simulink model "ThomasJana_WorkingCode (fix branch)"  (R2023a)
settings: Solver=FixedStepDiscrete  StartTime=0.0  StopTime=inf  FixedStep=0.0001  RelTol=1e-3
undefined symbols (not defined in the file): DiscIntNeverNeededParam
libraries: arduinolib x13, simulink x3, hdlsllib x2, slpidlib x1, mobileRoboticsTrainingLib x1, arduinosensorlib x1
(part 2 of 2)

== stateflow chart ThomasJana_WorkingCode (fix branch)/Motion Control1/Intersection Navigation V2 ==
  note: Basic Description
      | Default: Curve Navigation controls the velocity and angular velocity
      |
      | When infrared sensor 1 or 4 (IR1 and IR4) detect a black line, this Intersection Navigation subsystem takes control and calls the leftTurn or rightTurn procedure respectively.
      | Intersection procedure (same for both leftTurn or rightTurn):
      | 	Increment branchCounter to keep track of the number of branches.
      | 	Move forward a small distance to align with the turn.
      | 	Rotate in the correct direction until the middle two sensors detect a line again.
      | 	Pass control to Curve Navigation to navigate the offshoot.
      | 	If the offshoot comes to an end (all sensors detect white), rotate 180 degrees and navigate back to the main path.
      | 	If the offshoot ends in a detect line (all sensors detect black), stop, send a signal to the Object Detection subsystem to measure for an object, rotate 180 degrees and navigate back to the main path.
      | 		Add branch number from branchCounter to objectMap to indicate this branch has an object.
      | 	Pass control to Curve Navigation to navigate the offshoot returning to the main path.
      | 	When the peripheral sensors detect a black line again (meaning the robot has returned to the intersection with the main branch), control is passed to Intersection Navigation.
      | 	Move forward a small distance to align with the turn.
      | 	Rotate in the correct direction until the middle two sensors detect a line again.
      | 	Pass control back to Curve Navigation to continue traversing the main path.
      |
      | If all sensors detect black whilst the robot is on the main path, the endOfMaze procedure is called.
      | endOfMaze procedure:
      | 	Stop
      | 	Use objectMap to determine how many objects were discovered.
      | 	Find the branch number of the object with the smallest distance, saved to branchWithObject.
      | 		objectCounter provides number of object with smallest distance measured.
      | 		Obtain the n'th number in objectMap to determine the branch number containing said object (where n = objectCounter)
      | 	Invert branchWithObject such that it provides the number of the branch starting from the end of the maze.
      | 	Set renavigating to HIGH.
      |
      | Renavigating Procedure:
      | 	Rotate 180 degrees to re-traverse the maze.
      | 	set branchCounter to 0.
      | 	Pass control to Curve Navigation to renavigate maze.
      | 	If intersection is detected, increment branchCounter.
      | 	If branchCounter is equal to branchWithObject at an intersection, turn into that offshoot.
      | 	Pass control to Curve Navigation to navigate offshoot.
      | 	If all sensors detect black at the "detect object line", come to a stop.
  note: Note to self:
      | Make sure all blocks with forward velocity use curve-following algorithm (never move forward blindly)
      |
      | Neaten up blocks
      |
      | Add 4way navigation
      |
      | Make back and forth smaller (will need to be adjusted for real life speed)
  state analyseIntersection
    state returnToIntersection
      entry: distance0 = distance;
      state FollowTrack
        %middle two sense black
        velocity = -0.5;
        angular_velocity = 0;
      state TurnLeft
        entry:
        velocity = 0;
        angular_velocity = 2;
      state TurnRight
        entry:
        velocity = 0;
        angular_velocity = -2;
      (default) -> analyseIntersection.returnToIntersection.FollowTrack
      analyseIntersection.returnToIntersection.TurnRight -> analyseIntersection.returnToIntersection.FollowTrack : [IR3 == 0 && IR2 == 0]
      analyseIntersection.returnToIntersection.TurnLeft -> analyseIntersection.returnToIntersection.FollowTrack : [IR3 == 0 && IR2 == 0]
      analyseIntersection.returnToIntersection.FollowTrack -> analyseIntersection.returnToIntersection.TurnRight [order 2] : [IR2 == 1]
      analyseIntersection.returnToIntersection.FollowTrack -> analyseIntersection.returnToIntersection.TurnLeft [order 1] : [IR3 == 1]
    state moveForward
      entry: distance0 = distance;
      state FollowTrack
        %middle two sense black
        velocity = 1;
        angular_velocity = 0;
      state TurnLeft
        entry:
        velocity = 0;
        angular_velocity = -2;
      state TurnRight
        entry:
        velocity = 0;
        angular_velocity = 2;
      analyseIntersection.moveForward.FollowTrack -> analyseIntersection.moveForward.TurnLeft [order 1] : [IR3 == 1]
      analyseIntersection.moveForward.TurnRight -> analyseIntersection.moveForward.FollowTrack : [IR3 == 0 && IR2 == 0]
      analyseIntersection.moveForward.FollowTrack -> analyseIntersection.moveForward.TurnRight [order 2] : [IR2 == 1]
      analyseIntersection.moveForward.TurnLeft -> analyseIntersection.moveForward.FollowTrack : [IR3 == 0 && IR2 == 0]
      (default) -> analyseIntersection.moveForward.FollowTrack
    state chooseIntersectionType
      %left turn
      %extreme left turn
      %right turn
      %extreme right turn
      %end of maze
      %4-way junction
      entry: velocity = 0;
      angular_velocity = 0;
    state commenceIntersectionControl
      entry: velocity = 0;
    (default) -> analyseIntersection.moveForward
    chooseIntersectionType -> returnToIntersection [order 1] : [(IR2 == 0 || IR3 == 0)]
    returnToIntersection -> commenceIntersectionControl : [IR1 == 0 || IR4 == 0]
    (junction 486) -> returnToIntersection : {finishMaze = 1;}
    analyseIntersection.moveForward -> chooseIntersectionType : [IR1 == 1 && IR4 == 1]
    chooseIntersectionType -> (junction 486) [order 3] : [IR1 + IR2 + IR3 + IR4 == 4]{fourWay = 0;}
    chooseIntersectionType -> (junction 486) [order 2] : [IR1 + IR2 + IR3 + IR4 == 0]{fourWay = 0;}
  note: if fourway doesn't work now:
      | have it pick up if another intersection is ever picked up in the slight move forward, and then limit forward movement massivly.
      | If another interesction in opposite direction was ever picked up - four way
  state endOfMaze
    %procedure to locate position of closest object once maze is completed
    entry: velocity = 0;
    angular_velocity = 0;
    num = objectMap;
    while num > 0
    len = len + 1;
    num = fix(num/10);
    end
    branchWithObject = mod(fix(objectMap/10^(len - objectCounter)), 10);
    branchWithObject = branchCounter - branchWithObject + 1
    exit:
    renavigating = 1;
  state fullRotation
    %rotate 180 degrees to renavigate maze
    entry: phi0 = phi;
    during:
    velocity = 0;
    angular_velocity = -1;
  note: if fullInter == 1:
      | if all black:
  state followMain
    state TurnRight
      entry:
      velocity = 0;
      angular_velocity = 2;
    state FollowTrack
      %middle two sense black
      velocity = 1;
      angular_velocity = 0;
    state TurnLeft
      entry:
      velocity = 0;
      angular_velocity = -2;
    (default) -> followMain.FollowTrack
    followMain.FollowTrack -> followMain.TurnLeft [order 2] : [IR3 == 1]
    followMain.TurnRight -> followMain.FollowTrack : [IR3 == 0 && IR2 == 0]
    followMain.TurnLeft -> followMain.FollowTrack : [IR3 == 0 && IR2 == 0]
    followMain.FollowTrack -> followMain.TurnRight [order 4] : [IR2 == 1]
    (junction 442) -> followMain.FollowTrack
    (junction 440) -> followMain.FollowTrack
  state Wait
  state leftTurn
    %procedure for navigating an offshoot to the right of the main path
    state Rotate
      entry:  branchCounter = branchCounter +1
      state moveForward
        entry: velocity = 1;
      state rotateOffPath
        entry:
        velocity = 0;
        angular_velocity = -1;
      state rotateOntoPath
      (default) -> leftTurn.Rotate.moveForward
      leftTurn.Rotate.moveForward -> leftTurn.Rotate.rotateOffPath : [IR1 == 1]
      leftTurn.Rotate.rotateOffPath -> (junction 365) : [IR2 == 1 && IR3 == 1]
      (junction 365) -> leftTurn.Rotate.rotateOntoPath
    state returnToMain
      state FollowTrack
        %middle two sense black
        velocity = 1;
        angular_velocity = 0;
      state TurnRight
        entry:
        velocity = 0;
        angular_velocity = 2;
      state TurnLeft1
        entry:
        velocity = 0;
        angular_velocity = -2;
      (default) -> leftTurn.returnToMain.FollowTrack
      (junction 469) -> leftTurn.returnToMain.FollowTrack
      (junction 472) -> leftTurn.returnToMain.FollowTrack
      TurnLeft1 -> (junction 469) : [IR3 == 0 && IR2 == 0]
      leftTurn.returnToMain.TurnRight -> (junction 472) : [IR3 == 0 && IR2 == 0]
      leftTurn.returnToMain.FollowTrack -> (junction 471) [order 2] : [IR2 == 1]
      leftTurn.returnToMain.FollowTrack -> (junction 470) [order 1] : [IR3 == 1]
      (junction 471) -> leftTurn.returnToMain.TurnRight
      (junction 470) -> TurnLeft1
    state leftToMain
      state moveForward
        entry: velocity = 1;
      state rotateOntoPath
      state rotateOffPath
        entry:
        velocity = 0;
        angular_velocity = 1;
      (default) -> leftTurn.leftToMain.moveForward
      leftTurn.leftToMain.moveForward -> leftTurn.leftToMain.rotateOffPath : [IR1 == 1]
      (junction 393) -> leftTurn.leftToMain.rotateOntoPath
      leftTurn.leftToMain.rotateOffPath -> (junction 393) : [IR2 == 1 && IR3 == 1]
    state navigateOffshoot
      state FollowTrack
        %middle two sense black
        velocity = 1;
        angular_velocity = 0;
      state TurnLeft
        entry:
        velocity = 0;
        angular_velocity = -2;
      state TurnRight
        entry:
        velocity = 0;
        angular_velocity = 2;
      (default) -> leftTurn.navigateOffshoot.FollowTrack
      leftTurn.navigateOffshoot.FollowTrack -> (junction 460) [order 2] : [IR2 == 1]
      (junction 460) -> leftTurn.navigateOffshoot.TurnRight
      leftTurn.navigateOffshoot.FollowTrack -> (junction 463) [order 1] : [IR3 == 1]
      (junction 463) -> leftTurn.navigateOffshoot.TurnLeft
      (junction 461) -> leftTurn.navigateOffshoot.FollowTrack : [IR3 == 0 && IR2 == 0]
      (junction 462) -> leftTurn.navigateOffshoot.FollowTrack
      leftTurn.navigateOffshoot.TurnRight -> (junction 461)
      leftTurn.navigateOffshoot.TurnLeft -> (junction 462) : [IR3 == 0 && IR2 == 0]
    state fullRotation
      %rotate 180 degrees
      entry: phi0 = phi;
      during:
      velocity = 0;
      angular_velocity = -4;
    state stopAndMeasure
      entry:
      velocity = 0;
      angular_velocity = 0;
      collectMeasurement = 1;
      exit:
      collectMeasurement = 0;
    state finalStop
      velocity = 0;
      angular_velocity = 0;
    (default) -> leftTurn.Rotate
    leftTurn.Rotate.rotateOntoPath -> leftTurn.navigateOffshoot : [IR2 == 0]
    leftTurn.returnToMain -> leftToMain : [IR1 == 0]
    leftTurn.fullRotation -> leftTurn.returnToMain : [abs(phi - phi0) > 2.793 && abs(phi - phi0) < 3.491 && IR2 == 0 && IR3 == 0]
    leftTurn.navigateOffshoot -> (junction 263) [order 2]
    (junction 263) -> (junction 264) : [IR1 + IR2 + IR3 + IR4 == 0 && renavigating == 1]
    leftTurn.navigateOffshoot -> (junction 216) [order 1] : [IR1 == 1 && IR2 == 1 && IR3 == 1 && IR4 == 1]
    (junction 216) -> leftTurn.fullRotation
    leftTurn.navigateOffshoot -> leftTurn.stopAndMeasure [order 3] : [IR1 == 0 && IR2 == 0 && IR3 == 0 && IR4 ==0]{objectMap = objectMap*10 + branchCounter;} %detect or stop line
    leftTurn.stopAndMeasure -> leftTurn.fullRotation : after(1, sec) [measurementComplete == 1]
    (junction 264) -> leftTurn.finalStop
  state rightTurn
    %procedure for navigating an offshoot to the right of the main path
    state returnToMain
      state FollowTrack
        %middle two sense black
        velocity = 1;
        angular_velocity = 0;
      state TurnLeft
        entry:
        velocity = 0;
        angular_velocity = -2;
      state TurnRight
        entry:
        velocity = 0;
        angular_velocity = 2;
      (default) -> rightTurn.returnToMain.FollowTrack
      rightTurn.returnToMain.FollowTrack -> rightTurn.returnToMain.TurnRight [order 2] : [IR2 == 1]
      rightTurn.returnToMain.TurnRight -> rightTurn.returnToMain.FollowTrack : [IR3 == 0 && IR2 == 0]
      rightTurn.returnToMain.FollowTrack -> rightTurn.returnToMain.TurnLeft [order 1] : [IR3 == 1]
      rightTurn.returnToMain.TurnLeft -> rightTurn.returnToMain.FollowTrack : [IR3 == 0 && IR2 == 0]
    state Rotate
      entry:  branchCounter = branchCounter +1
      state moveForward
        entry: velocity = 1;
      state rotateOffPath
        entry:
        velocity = 0;
        angular_velocity = 1;
      state rotateOntoPath
      (default) -> rightTurn.Rotate.moveForward
      rightTurn.Rotate.moveForward -> rightTurn.Rotate.rotateOffPath : [IR4 == 1]
      rightTurn.Rotate.rotateOffPath -> (junction 311) : [IR2 == 1 && IR3 == 1]
      (junction 311) -> rightTurn.Rotate.rotateOntoPath
    state rightToMain
      %turn right back onto the main path
      state moveForward
        entry: velocity = 1;
      state rotateOffPath
        entry:
        velocity = 0;
        angular_velocity = 1;
      state rotateOntoPath
      (default) -> rightTurn.rightToMain.moveForward
      rightTurn.rightToMain.moveForward -> rightTurn.rightToMain.rotateOffPath : [IR4 == 1]
      rightTurn.rightToMain.rotateOffPath -> (junction 357) : [IR2 == 1 && IR3 == 1]
      (junction 357) -> rightTurn.rightToMain.rotateOntoPath
    state navigateOffshoot
      state FollowTrack
        %middle two sense black
        velocity = 1;
        angular_velocity = 0;
      state TurnLeft
        entry:
        velocity = 0;
        angular_velocity = -2;
      state TurnRight1
        entry:
        velocity = 0;
        angular_velocity = 2;
      rightTurn.navigateOffshoot.FollowTrack -> (junction 448) [order 2] : [IR2 == 1]
      rightTurn.navigateOffshoot.FollowTrack -> (junction 454) [order 1] : [IR3 == 1]
      (junction 448) -> TurnRight1
      (junction 454) -> rightTurn.navigateOffshoot.TurnLeft
      (junction 450) -> rightTurn.navigateOffshoot.FollowTrack
      (default) -> rightTurn.navigateOffshoot.FollowTrack
      (junction 452) -> rightTurn.navigateOffshoot.FollowTrack
      TurnRight1 -> (junction 450) : [IR3 == 0 && IR2 == 0]
      rightTurn.navigateOffshoot.TurnLeft -> (junction 452) : [IR3 == 0 && IR2 == 0]
    state stopAndMeasure
      entry:
      velocity = 0;
      angular_velocity = 0;
      collectMeasurement = 1;
      exit:
      collectMeasurement = 0;
    state fullRotation
      %rotate 180 degrees
      entry: phi0 = phi;
      during:
      velocity = 0;
      angular_velocity = -4;
    state finalStop
      velocity = 0;
      angular_velocity = 0;
    (default) -> rightTurn.Rotate
    rightTurn.returnToMain -> rightToMain : [IR4 == 0]
    rightTurn.fullRotation -> rightTurn.returnToMain : [abs(phi - phi0) > 2.793 && abs(phi - phi0) < 3.491 && IR2 == 0 && IR3 == 0]
    rightTurn.Rotate.rotateOntoPath -> rightTurn.navigateOffshoot : [IR3 == 0]
    rightTurn.navigateOffshoot -> (junction 254) [order 1]
    (junction 254) -> (junction 256) : [IR1 + IR2 + IR3 + IR4 == 0 && renavigating == 1]
    rightTurn.navigateOffshoot -> (junction 194) [order 3] : [IR1 == 1 && IR2 == 1 && IR3 == 1 && IR4 == 1]
    (junction 194) -> rightTurn.fullRotation
    rightTurn.navigateOffshoot -> rightTurn.stopAndMeasure [order 2] : [IR1 == 0 && IR2 == 0 && IR3 == 0 && IR4 ==0]{objectMap = objectMap*10 + branchCounter;} %detect or stop line
    rightTurn.stopAndMeasure -> rightTurn.fullRotation : after(1, sec) [measurementComplete == 1]
    (junction 256) -> rightTurn.finalStop
  state renavigatingCounter
    entry:
    branchCounter = branchCounter + 1;
  commenceIntersectionControl -> endOfMaze [order 2] : [finishMaze == 1]
  endOfMaze -> fullRotation : {branchCounter = 0;}
  commenceIntersectionControl -> (junction 481) [order 1] : [IR4 == 0]
  commenceIntersectionControl -> (junction 477) [order 3] : [IR1 == 0]
  (junction 481) -> rightTurn
  (junction 477) -> leftTurn
  fullRotation -> Wait : [IR2 == 1 && IR3 == 1]
  (junction 483) -> endOfMaze [commented out]
  followMain.FollowTrack -> analyseIntersection [order 3] : [renavigating == 0 && (IR1 == 0 || IR4 == 0)]
  followMain.FollowTrack -> analyseIntersection [order 1] : [IR1 == 0 && IR4 == 0 && renavigating == 0]{fourWay = 1;}
  (default) -> followMain
  followMain -> (junction 483) [commented out] : [IR1 + IR2 + IR3 + IR4 == 0]
  Wait -> followMain : [IR2 == 0 && IR3 == 0]
  (junction 446) -> (junction 442)
  (junction 444) -> (junction 440)
  renavigatingCounter -> followMain [order 1] : [IR1 == 1 && IR4 == 1]
  followMain -> renavigatingCounter : [(IR1 == 0 || IR4 == 0) && renavigating == 1]
  renavigatingCounter -> leftTurn.Rotate [order 2] : [IR1 == 0 && branchCounter == branchWithObject]
  leftTurn.leftToMain.rotateOntoPath -> (junction 446) : [IR2 == 0 && IR3 == 0]
  renavigatingCounter -> rightTurn.Rotate [order 3] : [IR4 == 0 && branchCounter == branchWithObject]
  rightTurn.rightToMain.rotateOntoPath -> (junction 444) [order 2] : [IR3 == 0 && IR2 == 0]
  rightTurn.rightToMain.rotateOntoPath -> (junction 498) [order 1] : [fourWay == 1]
  (junction 498) -> leftTurn : {fourWay = 0;}
  data: len local =0; num local =0; velocity output; angular_velocity output; IR1 input; IR2 input; IR3 input; IR4 input; collectMeasurement output; phi input; phi0 local; distance input; distance0 local =0; objectCounter input; objectMap output =0; branchCounter local =0; branchWithObject local =0; renavigating local =0; measurementComplete input; finishMaze local =0; fourWay local =0

== stateflow chart ThomasJana_WorkingCode (fix branch)/Motion Control1/LFRB Priority ==
  note: Basic Description
      | Default: Curve Navigation controls the velocity and angular velocity
      |
      | When infrared sensor 1 or 4 (IR1 and IR4) detect a black line, this Intersection Navigation subsystem takes control and calls the leftTurn or rightTurn procedure respectively.
      | Intersection procedure (same for both leftTurn or rightTurn):
      | 	Increment branchCounter to keep track of the number of branches.
      | 	Move forward a small distance to align with the turn.
      | 	Rotate in the correct direction until the middle two sensors detect a line again.
      | 	Pass control to Curve Navigation to navigate the offshoot.
      | 	If the offshoot comes to an end (all sensors detect white), rotate 180 degrees and navigate back to the main path.
      | 	If the offshoot ends in a detect line (all sensors detect black), stop, send a signal to the Object Detection subsystem to measure for an object, rotate 180 degrees and navigate back to the main path.
      | 		Add branch number from branchCounter to objectMap to indicate this branch has an object.
      | 	Pass control to Curve Navigation to navigate the offshoot returning to the main path.
      | 	When the peripheral sensors detect a black line again (meaning the robot has returned to the intersection with the main branch), control is passed to Intersection Navigation.
      | 	Move forward a small distance to align with the turn.
      | 	Rotate in the correct direction until the middle two sensors detect a line again.
      | 	Pass control back to Curve Navigation to continue traversing the main path.
      |
      | If all sensors detect black whilst the robot is on the main path, the endOfMaze procedure is called.
      | endOfMaze procedure:
      | 	Stop
      | 	Use objectMap to determine how many objects were discovered.
      | 	Find the branch number of the object with the smallest distance, saved to branchWithObject.
      | 		objectCounter provides number of object with smallest distance measured.
      | 		Obtain the n'th number in objectMap to determine the branch number containing said object (where n = objectCounter)
      | 	Invert branchWithObject such that it provides the number of the branch starting from the end of the maze.
      | 	Set renavigating to HIGH.
      |
      | Renavigating Procedure:
      | 	Rotate 180 degrees to re-traverse the maze.
      | 	set branchCounter to 0.
      | 	Pass control to Curve Navigation to renavigate maze.
      | 	If intersection is detected, increment branchCounter.
      | 	If branchCounter is equal to branchWithObject at an intersection, turn into that offshoot.
      | 	Pass control to Curve Navigation to navigate offshoot.
      | 	If all sensors detect black at the "detect object line", come to a stop.
  note: Note to self:
      | Make sure all blocks with forward velocity use curve-following algorithm (never move forward blindly)
      |
      | Neaten up blocks
      |
      | Add 4way navigation
      |
      | Make back and forth smaller (will need to be adjusted for real life speed)
  note: if fourway doesn't work now:
      | have it pick up if another intersection is ever picked up in the slight move forward, and then limit forward movement massivly.
      | If another interesction in opposite direction was ever picked up - four way
  state findObjects [commented out]
    velocity = 0;
    angular_velocity = 0;
  state startingConditions [commented out]
    entry: x0 = x;
    y0 = y;
  note: First thing to try: increase sampling time!
  state lineFollowing1
    entry:
    debuggingLightON =0;
    if onBranch == 0
    debuggingLightON = 0;
    end
    state allWhiteRotate
      entry: velocity = 0;
      phi0 = phi;
      angular_velocity = minorTurnDirection * -1;
    state ohShitRight
      angular_velocity = 1;
    state ohShitLeft
      angular_velocity = -1;
    state FollowTrack
      %middle two sense black
      velocity = 0.3;
      angular_velocity = 0;
    state TurnRight
      entry:
      phi0 = phi;
      velocity = 0;
      angular_velocity = 1;
      minorTurnDirection = -1;
      exit:
      if abs(phi0 - phi) >= 2.09
      turnAround = 1;
      end
      angular_velocity = 0;
    state TurnLeft
      entry:
      phi0 = phi;
      velocity = 0;
      angular_velocity = -1;
      minorTurnDirection = 1;
      exit:
      if abs(phi0 - phi) >= 2.09
      turnAround = 1;
      end
      angular_velocity = 0;
    allWhiteRotate -> ohShitRight [order 2] : [IR4 == 0 && onBranch == 0]
    allWhiteRotate -> ohShitLeft [order 3] : [IR1 == 0 && onBranch == 0]
    ohShitRight -> (junction 1028)
    ohShitLeft -> (junction 1028)
    lineFollowing1.FollowTrack -> allWhiteRotate [order 3] : [IR1 + IR2 + IR3 + IR4 == 4]
    allWhiteRotate -> (junction 1028) [order 1] : [IR2 == 0 && IR3 == 0]
    (junction 1028) -> lineFollowing1.FollowTrack [order 1] : [abs(phi - phi0) < 2.09]
    (junction 1028) -> lineFollowing1.FollowTrack [order 2] : [abs(phi - phi0) >= 2.09]{turnAround = 1;}
    (default) -> lineFollowing1.FollowTrack
    lineFollowing1.FollowTrack -> lineFollowing1.TurnLeft [order 1] : [IR3 == 1]
    lineFollowing1.TurnRight -> lineFollowing1.FollowTrack : [IR3 == 0 && IR2 == 0]
    lineFollowing1.FollowTrack -> lineFollowing1.TurnRight [order 2] : [IR2 == 1]
    lineFollowing1.TurnLeft -> lineFollowing1.FollowTrack : [IR3 == 0 && IR2 == 0]
  state lineFollowing [commented out]
    state FollowTrack [commented out]
      %middle two sense black
      velocity = 0.3;
      angular_velocity = 0;
    state TurnRight [commented out]
      entry:
      velocity = 0;
      angular_velocity = 1.5;
    state TurnLeft [commented out]
      entry:
      velocity = 0;
      angular_velocity = -1.5;
    (default) -> lineFollowing.FollowTrack [commented out]
    lineFollowing.FollowTrack -> lineFollowing.TurnLeft [commented out] : [IR3 == 1]
    lineFollowing.TurnRight -> lineFollowing.FollowTrack [commented out] : [IR3 == 0 && IR2 == 0]
    lineFollowing.TurnLeft -> lineFollowing.FollowTrack [commented out] : [IR3 == 0 && IR2 == 0]
    lineFollowing.FollowTrack -> lineFollowing.TurnRight [commented out] : [IR2 == 1]
  state turnRight1
    entry: lastTurn = 2;
    state moveForward
      entry: distance0 = distance;
      velocity = 1;
    state rotateOffPath
      %entry:
      %velocity = 0;
      %angular_velocity = 2;
    state rotateOntoPath
    state firstRotate
      entry:
      velocity = 0;
      angular_velocity = 2;
    (default) -> turnRight1.moveForward
    turnRight1.firstRotate -> turnRight1.rotateOffPath : [IR4 == 0]
    turnRight1.moveForward -> turnRight1.firstRotate : [IR4 == 1]
    turnRight1.rotateOffPath -> turnRight1.rotateOntoPath : [IR2 == 1 && IR3 == 1]
  state turnLeft1
    entry: lastTurn = 1;
    state rotateOffPath
      entry:
      velocity = 0;
      angular_velocity = -2;
    state moveForward
      entry: velocity = 1;
      distance0 = distance;
    state rotateOntoPath
    state firstRotate
      entry:
      velocity = 0;
      angular_velocity = -2;
    (default) -> turnLeft1.moveForward
    turnLeft1.moveForward -> turnLeft1.firstRotate : [IR1 == 1]
    turnLeft1.firstRotate -> turnLeft1.rotateOffPath : [IR1 == 0]
    turnLeft1.rotateOffPath -> (junction 854) : [IR2 == 1 && IR3 == 1]
    (junction 854) -> turnLeft1.rotateOntoPath
  state moveForward3
    entry: distance0 = distance;
    state forward
      %move forward to confirm what paths are available
      entry: velocity = 1;
      state leftBranch
        entry: leftBranch = 1;
      state default
      state rightBranch
        entry: rightBranch = 1;
      (default) -> default
      default -> rightBranch [order 1] : [IR4 == 0]
      default -> leftBranch [order 2] : [IR1 == 0]
      leftBranch -> rightBranch : [IR4 == 0]
      rightBranch -> leftBranch : [IR1 == 0]
    state chooseIntersection
      entry: velocity = 0;
      if leftBranch ==1
      debuggingLightON = 1;
      end
    (default) -> forward
    forward -> moveForward3.chooseIntersection : [abs(distance - distance0) >= 0.07]
  state turnRight [commented out]
    entry: steps = steps*10 + 3;
    state moveForward [commented out]
      entry: distance0 = distance;
      velocity = 1;
    state rotateOffPath [commented out]
      entry:
      velocity = 0;
      angular_velocity = 2;
    state rotateOntoPath [commented out]
    (default) -> turnRight.moveForward [commented out]
    turnRight.moveForward -> turnRight.rotateOffPath [commented out] : [IR4 == 1 && abs(distance - distance0) >= 0.04]
    turnRight.rotateOffPath -> turnRight.rotateOntoPath [commented out] : [IR2 == 1 && IR3 == 1]
  state turnLeft [commented out]
    entry: steps = steps*10 + 1;
    state rotateOffPath [commented out]
      entry:
      velocity = 0;
      angular_velocity = -2;
    state moveForward [commented out]
      entry: velocity = 1;
      distance0 = distance;
    state rotateOntoPath [commented out]
    (default) -> turnLeft.moveForward [commented out]
    turnLeft.moveForward -> turnLeft.rotateOffPath [commented out] : [abs(distance - distance0) >= 0.04 && IR1 == 1]
    turnLeft.rotateOffPath -> (junction 528) [commented out] : [IR2 == 1 && IR3 == 1]
    (junction 528) -> turnLeft.rotateOntoPath [commented out]
  state moveForward [commented out]
    state rightWiggle [commented out]
      entry: phi0 = phi;
      angular_velocity = 1;
      velocity = 0;
      during:
      if IR4 == 0
      rightBranch = 1;
      end
    state leftWiggle [commented out]
      entry: phi0 = phi;
      angular_velocity = -1;
      velocity = 0;
      during:
      if IR1 == 0
      leftBranch = 1;
      end
    state return1 [commented out]
      entry: phi0 = phi;
      angular_velocity = 1;
      during:
      if IR1 == 0
      leftBranch = 1;
      end
    state return2 [commented out]
      entry: phi0 = phi;
      angular_velocity = -1;
      during:
      if IR4 == 0
      rightBranch = 1;
      end
    state chooseIntersection [commented out]
      entry: angular_velocity = 0;
    (default) -> leftWiggle [commented out]
    leftWiggle -> return1 [commented out] : [abs(phi - phi0) >= 0.785]
    return1 -> (junction 819) [commented out] : [abs(phi - phi0) >= 1 && (IR2 == 0 || IR3 == 0)]
    (junction 819) -> rightWiggle [commented out] : after(1, sec)
    rightWiggle -> return2 [commented out] : [abs(phi - phi0) >= 0.785]
    (junction 821) -> moveForward.chooseIntersection [commented out] : after(1, sec)
    return2 -> (junction 821) [commented out] : [abs(phi - phi0) >= 1.17 && (IR2 == 0 || IR3 == 0)]
  state turnAround [commented out]
    entry: steps = steps*10 + 4;
    state moveForward [commented out]
      entry: distance0 = distance;
      velocity = 0.2;
    state Rotate [commented out]
      %rotate 180 degrees
      entry: phi0 = phi;
      during:
      velocity = 0;
      angular_velocity = -2;
    (default) -> turnAround.moveForward [commented out]
    turnAround.moveForward -> turnAround.Rotate [commented out] : [abs(distance0 - distance) >= 0.05]
  state allBlackDetected [commented out]
    %distinguish between the end of the maze and a detect line
    state moveForward [commented out]
      entry: distance0 = distance;
      velocity = 1;
    state confirmLineType [commented out]
      %if all sensors black - end of maze
      %else: detectObject
      entry: velocity = 0;
    (default) -> allBlackDetected.moveForward [commented out]
    allBlackDetected.moveForward -> confirmLineType [commented out] : %move 3 cm to check if line is thick or not
        | [abs(distance - distance0) >= 0.02]
  state endOfMaze
    branchfactor = -1;
    velocity = 0;
    angular_velocity = 0;
    %debuggingLightON = 1;
  state Rotate
    %rotate 180 degrees
    entry: phi0 = phi;
    during:
    velocity = 0;
    angular_velocity = -2;
  note: Figure out how to store array
  state blackLine [commented out]
    entry: velocity = 0;
    state moveForward_RightBranch [commented out]
      entry: distance0 = distance;
      state FollowTrack [commented out]
        %middle two sense black
        velocity = 0.3;
        angular_velocity = 0;
      state TurnRight [commented out]
        entry:
        velocity = 0;
        angular_velocity = 1.5;
      state TurnLeft [commented out]
        entry:
        velocity = 0;
        angular_velocity = -1.5;
      (default) -> blackLine.moveForward_RightBranch.FollowTrack [commented out]
      blackLine.moveForward_RightBranch.FollowTrack -> blackLine.moveForward_RightBranch.TurnLeft [commented out] : [IR3 == 1 && IR2 == 0]
      blackLine.moveForward_RightBranch.FollowTrack -> blackLine.moveForward_RightBranch.TurnRight [commented out] : [IR2 == 1 && IR3 == 0]
      blackLine.moveForward_RightBranch.TurnLeft -> blackLine.moveForward_RightBranch.FollowTrack [commented out] : [IR3 == 0 && IR2 == 0]
      blackLine.moveForward_RightBranch.TurnRight -> blackLine.moveForward_RightBranch.FollowTrack [commented out] : [IR3 == 0 && IR2 == 0]
    state moveForward1 [commented out]
      state FollowTrack [commented out]
        %middle two sense black
        velocity = 0.3;
        angular_velocity = 0;
      state TurnRight [commented out]
        entry:
        velocity = 0;
        angular_velocity = 1.5;
      state TurnLeft [commented out]
        entry:
        velocity = 0;
        angular_velocity = -1.5;
      (default) -> blackLine.moveForward1.FollowTrack [commented out]
      blackLine.moveForward1.FollowTrack -> blackLine.moveForward1.TurnLeft [commented out] : [IR3 == 1]
      blackLine.moveForward1.FollowTrack -> blackLine.moveForward1.TurnRight [commented out] : [IR2 == 1]
      blackLine.moveForward1.TurnRight -> blackLine.moveForward1.FollowTrack [commented out] : [IR3 == 0 && IR2 == 0]
      blackLine.moveForward1.TurnLeft -> blackLine.moveForward1.FollowTrack [commented out] : [IR3 == 0 && IR2 == 0]
    state selectIntersection [commented out]
      entry: velocity = 0;
    state moveForward_TJunction [commented out]
      %can't have line navigation for
      %a t-junction, as it starts rotating
      entry:distance0 = distance;
      velocity = 1;
      angular_velocity = 0;
    state detectObject [commented out]
      %if object, turn around
      %if no object, turn left back onto a path
    state stopAndMeasure [commented out]
    (default) -> moveForward_RightBranch [commented out]
    selectIntersection -> moveForward1 [commented out] : %if only a right branch and there is a forward section, continue moving forward
        | [leftBranch == 0 && rightBranch == 1 && (IR2 == 0 || IR3 == 0)]{rightBranch = 0;}
    moveForward_RightBranch -> (junction 749) [commented out]
    (junction 749) -> selectIntersection [commented out] : [abs(distance0 - distance) >= 0.04]
    (junction 825) -> (junction 749) [commented out]
    selectIntersection -> blackLine.detectObject [commented out] : %if line detected, check for an object
        | [leftBranch == 1 && rightBranch == 1]
    selectIntersection -> (junction 735) [commented out] : %if only right branch and no forward path, turn right
        | [leftBranch== 0 && rightBranch == 1 && IR1 + IR2 + IR3 + IR4 == 4]
    selectIntersection -> (junction 751) [commented out] : %if all pick up black, robot is at end of maze
        | [IR1 + IR2 + IR3 + IR4 == 0]
    (junction 823) -> moveForward_TJunction [commented out]
    moveForward_TJunction -> (junction 825) [commented out]
    blackLine.detectObject -> stopAndMeasure [commented out] : after(2, sec) [objectDistance < 0.5]
  state detectObject
    state DoNothing
    state UpdateClosestObj
      debuggingLightON = 1;
      closestObj = objectDistance;
      returnBranch = branchNumber;
    (default) -> DoNothing
    DoNothing -> UpdateClosestObj : [(objectDistance < closestObj && objectDistance ~=0) || branchNumber == 1]
  state FoundHome
    debuggingLightON =0;
  state turnAround1
    entry:
    turnAround = 1;
    branchNumber = branchNumber + branchfactor;
    state moveForward
      entry: distance0 = distance;
      velocity = 0.2;
    state Rotate
      %rotate 180 degrees
      entry: phi0 = phi;
      during:
      velocity = 0;
      angular_velocity = -1;
    (default) -> turnAround1.moveForward
    turnAround1.moveForward -> turnAround1.Rotate : [abs(distance0 - distance) >= 0.05]
  (default) -> startingConditions [commented out]
  startingConditions -> lineFollowing [commented out]
  lineFollowing -> findObjects [commented out] : [renavigating == 1&& abs(x) <= 0.5 && abs(y) <= 0.5]
  (default) -> lineFollowing1
  (junction 664) -> lineFollowing [commented out] : [IR2 == 0 || IR3 == 0]
  turnLeft.rotateOntoPath -> (junction 664) [commented out]
  (junction 753) -> lineFollowing [commented out]
  turnRight.rotateOntoPath -> (junction 753) [commented out] : [IR2 == 0 || IR3 == 0]
  lineFollowing -> (junction 733) [commented out] : [IR1 + IR2 + IR3 + IR4 == 4]
  (junction 733) -> (junction 681) [commented out]
  (junction 829) -> lineFollowing [commented out]
  lineFollowing1 -> turnRight1 [commented out] : [IR4 == 0 && onBranch == 1 && lastTurn == 2]{onBranch = 0;}
  moveForward1 -> (junction 829) [commented out] : [IR4 == 1]
  lineFollowing1 -> turnLeft1 [commented out] : %If left detected, and currently returning to main branch and turned left onto that branch, turn left
      | [IR1 == 0 && onBranch == 1 && lastTurn == 1]{onBranch = 0;}
  (junction 683) -> lineFollowing [commented out] : [abs(phi - phi0) >= 2.51 &&  IR3 == 0]
  turnAround.Rotate -> (junction 683) [commented out]
  lineFollowing.FollowTrack -> moveForward [commented out] : [IR1 == 0 || IR4 == 0]
  turnLeft1.rotateOntoPath -> lineFollowing1 : %orientated onto a path
      | [IR2 == 0 && IR3 == 0]
  turnRight1.rotateOntoPath -> lineFollowing1 : [IR2 == 0 && IR3 == 0]
  Rotate -> lineFollowing1 : [abs(phi - phi0) >= 2 &&  IR3 == 0]
  lineFollowing1 -> moveForward3 [order 2] : [IR2 + IR3 + IR4 <=2 && IR1 == 0]{leftBranch = 1;}
  lineFollowing1 -> moveForward3 [order 1] : [IR1 + IR2 + IR3 <= 2 && IR4 == 0]{rightBranch = 1;}
  (junction 932) -> lineFollowing1 : [abs(phi - phi0) >= 2 &&  IR3 == 0]
  (junction 948) -> turnRight1
  (junction 898) -> turnRight1
  (junction 1015) -> turnRight1
  (junction 1013) -> turnLeft1
  (junction 900) -> turnLeft1
  (junction 950) -> turnLeft1
  (junction 667) -> turnLeft.rotateOffPath [commented out] : {leftBranch = 0; rightBranch = 0;}
  moveForward3.chooseIntersection -> (junction 900) [order 7] : [leftBranch == 1 && rightBranch == 0]{leftBranch = 0, onBranch = 1, branchNumber = branchNumber + branchfactor;}
  moveForward3.chooseIntersection -> (junction 948) [order 3] : [rightBranch == 1 && turnAround == 1 && lastTurn == 2]{onBranch = 0, rightBranch = 0, leftBranch = 0, turnAround = 0;}
  moveForward3.chooseIntersection -> (junction 1013) [order 5] : [IR1 + IR2 + IR3 + IR4 == 4 && leftBranch == 1 && rightBranch == 0]
  moveForward3.chooseIntersection -> (junction 898) [order 8] : [rightBranch == 1 && leftBranch == 0]{rightBranch = 0, onBranch = 1, branchNumber = branchNumber + branchfactor;}
  moveForward3.chooseIntersection -> (junction 1015) [order 6] : [IR1 + IR2 + IR3 + IR4 == 4 && rightBranch == 1 && leftBranch == 0]
  moveForward3.chooseIntersection -> (junction 950) [order 2] : [leftBranch == 1 && turnAround == 1 && lastTurn == 1]{leftBranch = 0, rightBranch = 0, onBranch = 0, turnAround = 0;}
  moveForward3.chooseIntersection -> detectObject [order 4] : [leftBranch == 1 && rightBranch == 1 && onBranch == 1 && turnAround == 0]
  moveForward3.chooseIntersection -> endOfMaze [order 1] : [IR1 + IR2 + IR3 + IR4 == 0 && onBranch == 0 && turnAround == 0] {leftBranch = 0, rightBranch = 0, debuggingLightON = 1;}%make sure this one is first execution priority
  (junction 827) -> turnAround.Rotate [commented out]
  moveForward.chooseIntersection -> turnLeft [commented out] : [leftBranch == 1 && rightBranch == 0]{leftBranch = 0;}
  endOfMaze -> Rotate
  moveForward.chooseIntersection -> (junction 823) [commented out] : [leftBranch == 1 && rightBranch == 1]
  moveForward.chooseIntersection -> blackLine [commented out] : [leftBranch == 0 && rightBranch == 1]
  (junction 737) -> turnRight [commented out]
  confirmLineType -> endOfMaze [commented out] : [IR1 + IR2 + IR3 + IR4 == 0]
  (junction 681) -> turnAround [commented out]
  confirmLineType -> detectObject [commented out] : [IR1 + IR2 + IR3 + IR4 ~= 0]
  (junction 674) -> turnAround [commented out]
  allBlackDetected -> detectObject [commented out] : [onBranch == 1]
  detectObject -> FoundHome [order 2] : [(branchNumber == returnBranch) &&(branchfactor== -1)]%[(objectDistance < closestObj+0.05|| objectDistance > closestObj-0.05) && branchfactor == -1]
  (junction 751) -> (junction 827) [commented out] : {renavigating = 1;}
  detectObject -> turnAround1.Rotate [order 1] : after(0.05,sec){turnAround = 1;} %add to branch counter and include 2 second time for measurement
  (junction 735) -> (junction 737) [commented out] : {rightBranch = 0;}
  turnAround1.Rotate -> (junction 932)
  blackLine.detectObject -> (junction 667) [commented out] : after(2, sec) [objectDistance > 0.5 || objectDistance == 0]
  stopAndMeasure -> (junction 674) [commented out] : after(0.5, sec)
  data: velocity output; angular_velocity output; IR1 input; IR2 input; IR3 input; IR4 input; phi input; phi0 local; distance input; distance0 local =0; turnAround local =0; objectDistance input; lastTurn local =0; leftBranch local =0; rightBranch local =0; closestObj local =0; branchNumber local =0; branchfactor local =1; returnBranch local =0; debuggingLightON output =0; minorTurnDirection local =0; onBranch local =0
